simulink model "Res_13"  (R2018b)
settings: Solver=ode4  StartTime=0.0  StopTime=1.8  FixedStep=0.0001  RelTol=1e-3  EnableMultiTasking=on
values from neighbouring files (symbols this model uses):
  b = 25    [result_13.m]
  k = 800    [result_13.m]
  m = 2    [result_13.m]
undefined symbols (not defined in the file or in its folder): sgn
settings Model: Creator=makha  LastModifiedBy=makha

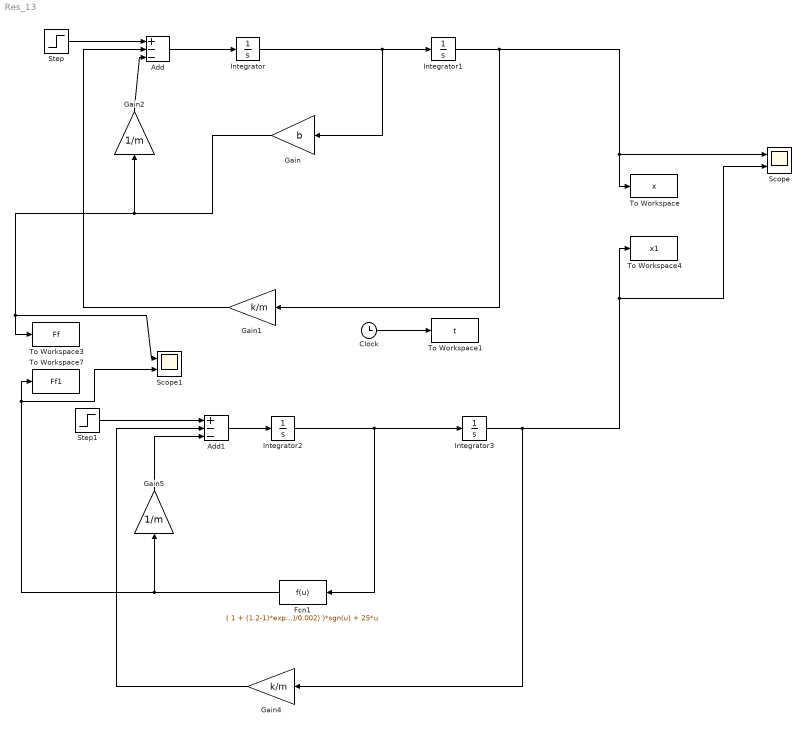
== system Res_13 ==
  Add : Sum  Inputs=+--
  Add1 : Sum  Inputs=+--
  Clock : Clock
  Fcn1 : Fcn  Expr=( 1 + (1.2-1)*exp(-abs(u)/0.002) )*sgn(u) + 25*u
  Gain : Gain  Gain=b
  Gain1 : Gain  Gain=k/m
  Gain2 : Gain  Gain=1/m
  Gain4 : Gain  Gain=k/m
  Gain5 : Gain  Gain=1/m
  Integrator{,1..3} (4 alike) : Integrator
  Scope : Scope  NumInputPorts=2
  Scope1 : Scope  NumInputPorts=2
  Step : Step  Time=0.2  After=15  SampleTime=0.0001
  Step1 : Step  Time=0.2  After=15  SampleTime=0.0001
  To Workspace : ToWorkspace  VariableName=x  SampleTime=-1
  To Workspace1 : ToWorkspace  VariableName=t  SampleTime=-1
  To Workspace3 : ToWorkspace  VariableName=Ff  SampleTime=-1
  To Workspace4 : ToWorkspace  VariableName=x1  SampleTime=-1
  To Workspace7 : ToWorkspace  VariableName=Ff1  SampleTime=-1
  wires:
  Step/1 -> Add/1
  Clock/1 -> To Workspace1/1
  Add/1 -> Integrator/1
  Integrator/1 -> Gain/1, Integrator1/1
  Integrator1/1 -> Gain1/1, Scope/1, To Workspace/1
  Gain1/1 -> Add/2
  Gain/1 -> To Workspace3/1, Scope1/1, Gain2/1
  Gain2/1 -> Add/3
  Fcn1/1 -> Scope1/2, To Workspace7/1, Gain5/1
  Gain5/1 -> Add1/3
  Gain4/1 -> Add1/2
  Integrator3/1 -> Scope/2, To Workspace4/1, Gain4/1
  Add1/1 -> Integrator2/1
  Step1/1 -> Add1/1
  Integrator2/1 -> Integrator3/1, Fcn1/1
